simulink model "adcs_full_loop"  (R2025a)
settings: Solver=ode45  StartTime=0.0  StopTime=800  RelTol=1e-8
settings Model: Creator=saipr  LastModifiedBy=saipr

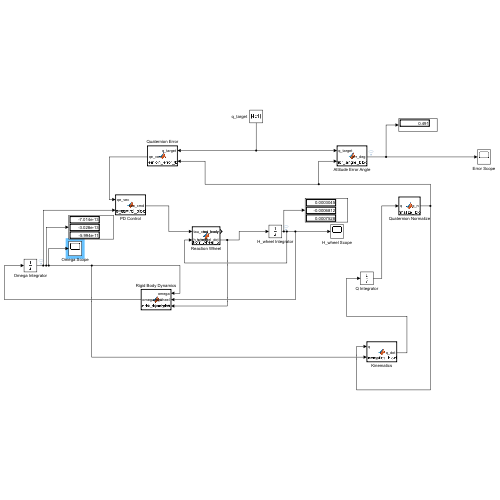
[thumbnail: Simulink's stored preview of the top-level diagram]
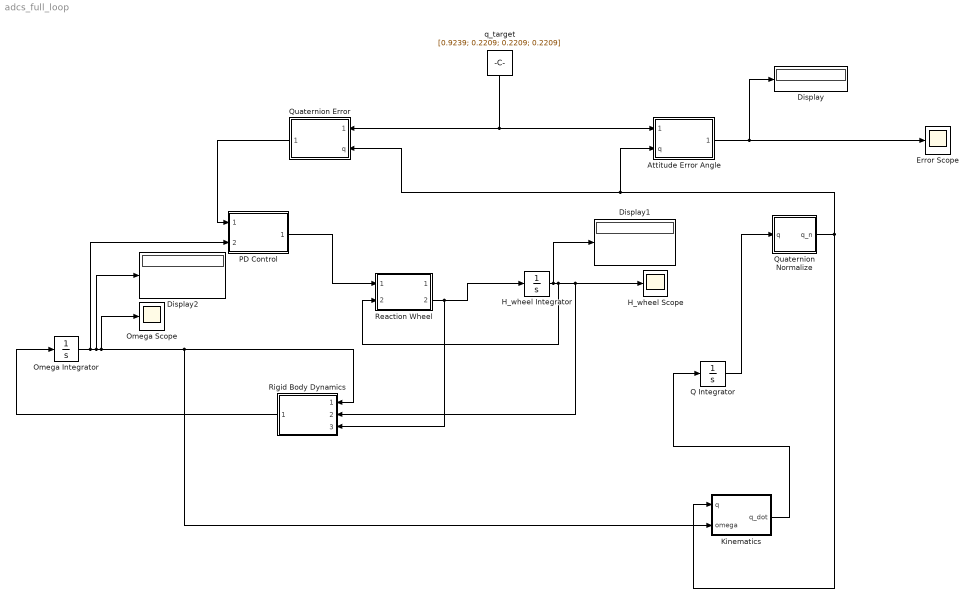
== system adcs_full_loop ==
  Attitude Error Angle : MATLAB Function  TreatAsAtomicUnit=on
  Display : Display
  Display1 : Display
  Display2 : Display
  Error Scope : Scope
      settings: ActiveDisplayYMinimum=-5.0718476498897909  ActiveDisplayYMaximum=50.556728377700132  DataLoggingVariableName=error_data
  H_wheel Integrator : Integrator  InitialCondition=[0; 0; 0]
  H_wheel Scope : Scope
      settings: ActiveDisplayYMinimum=-0.0026361710442873564  ActiveDisplayYMaximum=0.0011327382662079206  DataLoggingVariableName=h_wheel_data
  Kinematics : MATLAB Function  TreatAsAtomicUnit=on
  Omega Integrator : Integrator  InitialCondition=[0.02; -0.015; 0.025]
  Omega Scope : Scope
      settings: ActiveDisplayYMinimum=-0.023008799901616188  ActiveDisplayYMaximum=0.057079199114545683  DataLoggingVariableName=omega_data
  PD Control : MATLAB Function  TreatAsAtomicUnit=on
  Q Integrator : Integrator  InitialCondition=[1; 0; 0; 0]
  Quaternion Error : MATLAB Function  TreatAsAtomicUnit=on
  Quaternion Normalize : MATLAB Function  TreatAsAtomicUnit=on
  Reaction Wheel : MATLAB Function  TreatAsAtomicUnit=on
  Rigid Body Dynamics : MATLAB Function  TreatAsAtomicUnit=on
  q_target : Constant  Value=[0.9239; 0.2209; 0.2209; 0.2209]
  wires:
  q_target/1 -> Attitude Error Angle/1(q_target), Quaternion Error/1(q_target)
  Quaternion Normalize/1(q_n) -> Attitude Error Angle/2(q), Quaternion Error/2(q), Kinematics/1(q)
  Kinematics/1(q_dot) -> Q Integrator/1
  Q Integrator/1 -> Quaternion Normalize/1(q)
  Attitude Error Angle/1(err_deg) -> Display/1, Error Scope/1
  PD Control/1(tau_cmd) -> Reaction Wheel/1(tau_cmd_body)
  Quaternion Error/1(qe_vec) -> PD Control/1(qe_vec)
  H_wheel Integrator/1 -> Reaction Wheel/2(h_wheel), Rigid Body Dynamics/2(h_wheel), H_wheel Scope/1, Display1/1
  Reaction Wheel/2(h_wheel_dot) -> H_wheel Integrator/1, Rigid Body Dynamics/3(h_wheel_dot)
  Omega Integrator/1 -> PD Control/2(omega), Kinematics/2(omega), Rigid Body Dynamics/1(omega), Omega Scope/1, Display2/1
  Rigid Body Dynamics/1(omega_dot) -> Omega Integrator/1

== matlab function adcs_full_loop/Kinematics ==
  data: q input; q_dot output; omega input
function q_dot = kinematics_block(q, omega)
    wx = omega(1); wy = omega(2); wz = omega(3);
    Omega = [ 0 -wx -wy -wz; wx 0 wz -wy; wy -wz 0 wx; wz wy -wx 0 ];
    q_dot = 0.5 * Omega * q;
end

== matlab function adcs_full_loop/Reaction Wheel ==
  data: tau_cmd_body input; tau_body output; h_wheel input; h_wheel_dot output
function [tau_body, h_wheel_dot] = reaction_wheel_block(tau_cmd_body, h_wheel)
    h_max = 0.01; tau_max = 0.0006;   % same values as reaction_wheel_model.m
    tau_wheel_cmd = -tau_cmd_body;     % same sign fix as the debugged .m version
    tau_actual = zeros(3,1);
    for i = 1:3
        tau_actual(i) = max(min(tau_wheel_cmd(i), tau_max), -tau_max);
    end
    for i = 1:3
        if (h_wheel(i) >= h_max && tau_actual(i) > 0) || ...
           (h_wheel(i) <= -h_max && tau_actual(i) < 0)
            tau_actual(i) = 0;
        end
    end
    h_wheel_dot = tau_actual;
    tau_body = -tau_actual;
end

== matlab function adcs_full_loop/Quaternion Normalize ==
  data: q input; q_n output
function q_n = normalize_block(q)
    q_n = q / norm(q);
end

== matlab function adcs_full_loop/Attitude Error Angle ==
  data: q_target input; err_deg output; q input
function err_deg = error_angle_block(q_target, q)
    q0 = q(1); qv = q(2:4);
    r0 = q_target(1); rv = -q_target(2:4);
    qe0 = r0*q0 - dot(rv,qv);
    if qe0 < 0, qe0 = -qe0; end
    qe0 = min(max(qe0,-1),1);
    err_deg = 2*acosd(qe0);
end

== matlab function adcs_full_loop/Quaternion Error ==
  data: q_target input; qe_vec output; q input
function qe_vec = quaternion_error_block(q_target, q)
    q0 = q(1); qv = q(2:4);
    r0 = q_target(1); rv = -q_target(2:4);  % conjugate of q_target inline
    qe0 = r0*q0 - dot(rv,qv);
    qe_vec = r0*qv + q0*rv + cross(rv,qv);
    if qe0 < 0
        qe_vec = -qe_vec;   % shortest-path correction, same as pid_attitude_control.m
    end
end

== matlab function adcs_full_loop/PD Control ==
  data: qe_vec input; tau_cmd output; omega input
function tau_cmd = pd_control_block(qe_vec, omega)
    Kp = 3e-3;   % SAME gains as main_pointing.m -- keep in sync if you retune
    Kd = 1.2e-2;
    tau_cmd = -Kp*qe_vec - Kd*omega;
end

== matlab function adcs_full_loop/Rigid Body Dynamics ==
  data: omega input; omega_dot output; h_wheel input; h_wheel_dot input
function omega_dot = rigid_body_dynamics_block(omega, h_wheel, h_wheel_dot)
    I = diag([0.04187, 0.04187, 0.006667]);   % same 3U CubeSat inertia as inertia_properties.m
    H_total = I*omega + h_wheel;
    gyroscopic_term = cross(omega, H_total);
    omega_dot = I \ (-gyroscopic_term - h_wheel_dot);   % tau_ext = 0 (pointing loop only, no disturbance)
end
